simulink model "Mode_Logic_Ex"  (R2020b)
settings: Solver=FixedStepDiscrete  StartTime=0.0  StopTime=10  FixedStep=0.001  RelTol=1e-3  EnableMultiTasking=on
PreLoadFcn:
  | % Copyright 2011-2015 The MathWorks, Inc.
  | 
  | HEV_Model_HomeDir = pwd;
  | addpath(pwd);
  | 
  | load('Mode_Logic_data.mat');
CloseFcn:
  | rmpath(pwd);
settings Model: Creator=aroy  LastModifiedBy=rarora
settings SolverCC: NumberNewtonIterations=2
settings DataIOCC: LimitDataPoints=on  SaveOutput=off  SaveTime=off  ReturnWorkspaceOutputs=off
settings OptimizationCC: DefaultParameterBehavior=Inlined  LifeSpan=Inf  MaxStackSize=64  EfficientTunableParamExpr=on
settings DebuggingCC: AllowSymbolicDim=off  PregeneratedLibrarySubsystemCodeDiagnostic=none  SFUnexpectedBacktrackingDiag=warning  SFNoUnconditionalDefaultTransitionDiag=warning  SFExecutionAtInitializationDiag=none  ArithmeticOperatorsInVariantConditions=warning
settings ModelReferenceCC: PropagateSignalLabelsOutOfModel=off
settings SFSimCC: SimUseLocalCustomCode=off  MATLABDynamicMemAlloc=off  CustomCodeUndefinedFunction=UseInterfaceOnly
settings RTWCC: Description=Embedded Coder  SystemTargetFile=ert.tlc  GenCodeOnly=on  TemplateMakefile=ert_default_tmf  RTWUseLocalCustomCode=off
settings CodeAppCC: IgnoreCustomStorageClasses=off  StateflowObjectComments=on
settings ERTTargetCC: MultiwordLength=2048  SupportNonFinite=off  SupportComplex=off  ERTCustomFileTemplate=example_file_process.tlc  ConvertIfToSwitch=off  SuppressUnreachableDefaultCases=off
settings ConfigComp: CovMetricSettings=dw  CovSaveCumulativeToWorkspaceVar=on  CovSaveSingleToWorkspaceVar=on  CovExternalEMLEnable=off  DVModelCoverageObjectives=MCDC  DVTestSuiteOptimization=CombinedObjectives (Nonlinear Extended)  DVDetectDeadLogic=on  DVDetectActiveLogic=on  DVDetectIntegerOverflow=off  DVRebuildModelRepresentation=Always  PSVerificationMode=BugFinder  PSVerificationSettings=PrjConfigAndMisraC2012  PSResultDir=misrapsanalysis  PSAddSuffixToResultDir=on  PSModelRefVerifDepth=All  PSAutoStubLUT=on
settings SimscapeCC: SimscapeNormalizeSystem=off

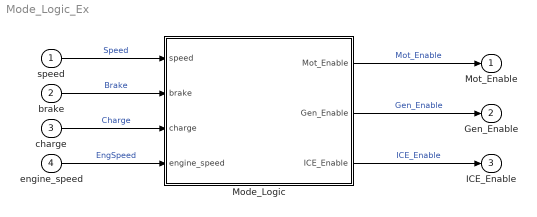
== system Mode_Logic_Ex ==
  speed : Inport  OutDataTypeStr=double  Unit=km/hr  PortDimensions=1  Interpolate=off
  brake : Inport  Port=2  OutDataTypeStr=double  PortDimensions=1  SampleTime=[0.001,0]
  charge : Inport  Port=3  OutMin=0  OutMax=100  OutDataTypeStr=double  PortDimensions=1  SampleTime=[0.001,0]  Interpolate=off
  engine_speed : Inport  Port=4  OutDataTypeStr=double  PortDimensions=1  SampleTime=[0.001,0]  Interpolate=off
  Mode_Logic : Stateflow chart  TreatAsAtomicUnit=on
  Mot_Enable : Outport  OutDataTypeStr=double  PortDimensions=1  SampleTime=[0.001,0]  VectorParamsAs1DForOutWhenUnconnected=off
  Gen_Enable : Outport  Port=2  OutDataTypeStr=double  PortDimensions=1  SampleTime=[0.001,0]  VectorParamsAs1DForOutWhenUnconnected=off
  ICE_Enable : Outport  Port=3  OutDataTypeStr=double  PortDimensions=1  SampleTime=[0.001,0]  VectorParamsAs1DForOutWhenUnconnected=off
  wires:
  speed/1 -> Mode_Logic/1(speed)  "Speed"
  brake/1 -> Mode_Logic/2(brake)  "Brake"
  charge/1 -> Mode_Logic/3(charge)  "Charge"
  engine_speed/1 -> Mode_Logic/4(engine_speed)  "EngSpeed"
  Mode_Logic/1(Mot_Enable) -> Mot_Enable/1  "Mot_Enable"
  Mode_Logic/2(Gen_Enable) -> Gen_Enable/1  "Gen_Enable"
  Mode_Logic/3(ICE_Enable) -> ICE_Enable/1  "ICE_Enable"

== stateflow chart Mode_Logic_Ex/Mode_Logic ==
  settings: updateMethod=DISCRETE
  state Motion_mode
    state Start_mode
      entry: Gen_Enable=1;
      Mot_Enable=1;
      ICE_Enable=0;
    state Normal_mode
      entry: ICE_Enable=1;
      state Accelerate_mode
        entry: Gen_Enable=0;
        Mot_Enable=1;
      state Cruise_mode
        entry: Mot_Enable=1;
        state charge
          entry:Gen_Enable=1;
          Mot_Enable = 0;
        state nocharge
          entry:Gen_Enable=0;
        (default) -> nocharge
        charge -> nocharge : [charge>=100]
        nocharge -> charge : [charge<30]
      (default) -> Accelerate_mode
      Cruise_mode -> Accelerate_mode : [(speed <0.998*oldspeed() ...
          | || speed>1.002*oldspeed()) ...
          | && charge>=32]
      Accelerate_mode -> Cruise_mode : [(speed >0.998*oldspeed() ...
          |  && speed<1.002* ...
          | oldspeed())|| charge<=30]
    (default) -> Start_mode
    Normal_mode -> Start_mode : [engine_speed<=EngOffRPM]
    Start_mode -> Normal_mode : [engine_speed>EngOnRPM]
  state Brake_mode
    entry: Mot_Enable=1;
    Gen_Enable=0;
    ICE_Enable=0;
  (default) -> Motion_mode
  Motion_mode -> Brake_mode : [brake>=0.05]
  Brake_mode -> Motion_mode : [brake<0.05]
  data: y function_output double; speed input; Mot_Enable output; Gen_Enable output; brake input; speed_buffer local double size=21; ICE_Enable output; charge input; engine_speed input; EngOnRPM constant double =HEV_Param.Control.Engine_Start_RPM; EngOffRPM constant double =HEV_Param.Control.Engine_Stop_RPM
  function y = oldspeed:
    | function y = oldspeed
    | speed_buffer(2:end) = speed_buffer(1:end-1);
    | speed_buffer(1) = speed;
    | y = mean(speed_buffer);
